simulink model "SimulationTest"  (R2025a)
settings: Solver=ode45  StartTime=0.0  StopTime=100  FixedStep=0.01  MaxStep=0.01  MinStep=0.001  RelTol=1e-3
model workspace (MAT data in the model file):
  L = 0.25
  R = 0.05
libraries: simulink x3, slpidlib x1
settings Model: PacingRate=1000  Creator=levirogalla  LastModifiedBy=levirogalla

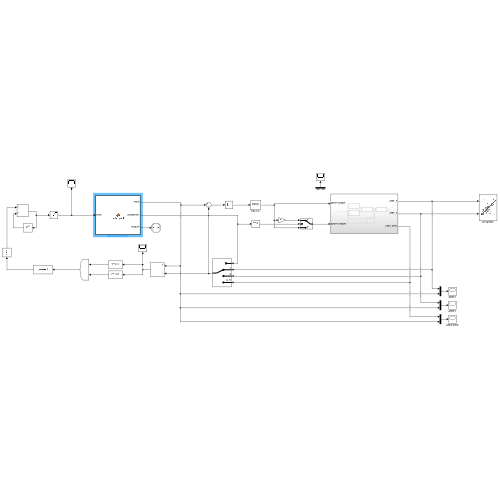
[thumbnail: Simulink's stored preview of the top-level diagram]
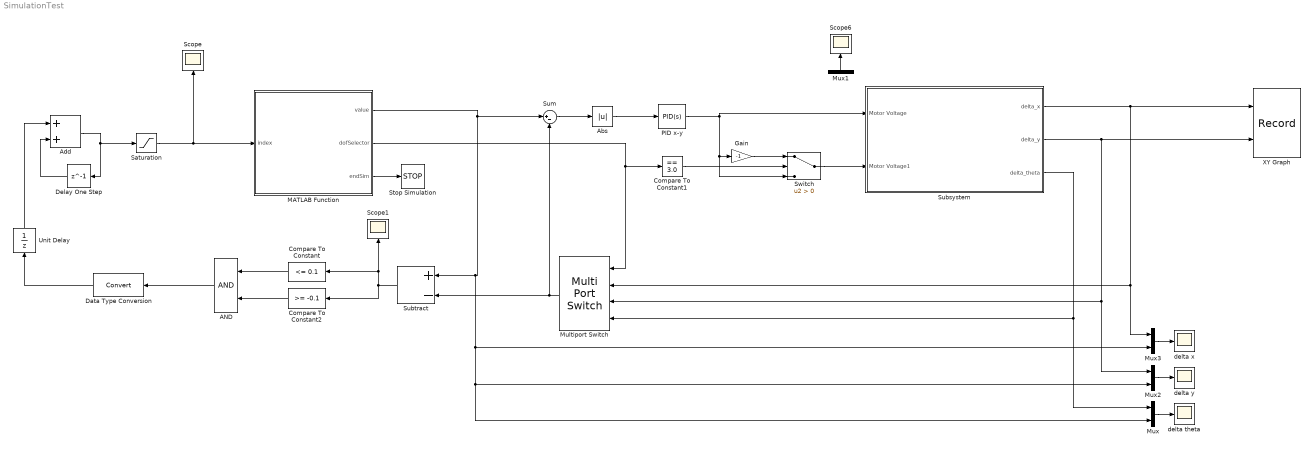
== system SimulationTest ==
  AND : Logic  IconShape=distinctive  AllPortsSameDT=off  OutDataTypeStr=boolean
  Abs : Abs  SaturateOnIntegerOverflow=off
  Add : Sum
  Compare To Constant : simulink/Logic and Bit Operations/Compare To Constant  relop=<=  const=0.1  OutDataTypeStr=boolean
  Compare To Constant1 : simulink/Logic and Bit Operations/Compare To Constant  relop===  const=3.0  OutDataTypeStr=boolean
  Compare To Constant2 : simulink/Logic and Bit Operations/Compare To Constant  relop=>=  const=-0.1  OutDataTypeStr=boolean
  Data Type Conversion : DataTypeConversion  SaturateOnIntegerOverflow=off  RndMeth=Floor
  Delay One Step : Delay  DelayLength=1
  Gain : Gain  Gain=-1
  MATLAB Function : MATLAB Function  TreatAsAtomicUnit=on
  Multiport Switch : MultiPortSwitch  SaturateOnIntegerOverflow=off  InputSameDT=off
  Mux{,1..3} (4 alike) : Mux  Inputs=2
  PID x-y : slpidlib/PID Controller  Controller=PID  Form=Parallel  TimeDomain=Continuous-time  UseExternalTs=off  SampleTime=-1  IntegratorMethod=Forward Euler  FilterMethod=Forward Euler  ControllerParametersSource=internal  P=0.25  I=0.001  UseKiTs=off  D=6.25  UseExternalDerivativeSource=off  N=100  UseFilter=on  TunerSelectOption=Transfer Function Based (PID Tuner App)  InitialConditionSource=internal  InitialConditionForIntegrator=0  InitialConditionForFilter=0  DifferentiatorICPrevScaledInput=0  ExternalReset=none  TrackingMode=off  Kt=1  LimitOutput=off  SatLimitsSource=internal  UpperSaturationLimit=50  LowerSaturationLimit=-inf  LinearizeAsGain=on  AntiWindupMode=none  Kb=1  LimitIntegrator=off  UpperIntegratorSaturationLimit=inf  LowerIntegratorSaturationLimit=-inf  POutMin=[]  POutMax=[]  IOutMin=[]  IOutMax=[]  DOutMin=[]  DOutMax=[]  NOutMin=[]  NOutMax=[]  SumOutMin=[]  SumOutMax=[]  SaturationOutMin=[]  SaturationOutMax=[]  PParamMin=[]  PParamMax=[]  IParamMin=[]  IParamMax=[]  DParamMin=[]  DParamMax=[]  NParamMin=[]  NParamMax=[]  KbParamMin=[]  KbParamMax=[]  KtParamMin=[]  KtParamMax=[]  KbOutMin=[]  KbOutMax=[]  KtOutMin=[]  KtOutMax=[]  IntegratorOutMin=[]  IntegratorOutMax=[]  FilterOutMin=[]  FilterOutMax=[]  SumI1OutMin=[]  SumI1OutMax=[]  SumI2OutMin=[]  SumI2OutMax=[]  SumI3OutMin=[]  SumI3OutMax=[]  SumI4OutMin=[]  SumI4OutMax=[]  SumDOutMin=[]  SumDOutMax=[]  DifferentiatorOutMin=[]  DifferentiatorOutMax=[]  FilterDiffOutCoefMin=[]  FilterDiffOutCoefMax=[]  ReciprocalOutMin=[]  ReciprocalOutMax=[]  SumDenOutMin=[]  SumDenOutMax=[]  SumNumOutMin=[]  SumNumOutMax=[]  DivideOutMin=[]  DivideOutMax=[]  UdiffTsProdOutMin=[]  UdiffTsProdOutMax=[]  NTsProdOutMin=[]  NTsProdOutMax=[]  UintegralTsProdOutMin=[]  UintegralTsProdOutMax=[]  UngainTsProdOutMin=[]  UngainTsProdOutMax=[]  ClampingZeroOutDataTypeStr=Inherit: Inherit via back propagation  ClampingZeroOutMin=[]  ClampingZeroOutMax=[]  FilterDenConstantOutDataTypeStr=Inherit: Inherit via back propagation  FilterDenConstantOutMin=[]  FilterDenConstantOutMax=[]  PCopyOutDataTypeStr=Inherit: Inherit via back propagation  PCopyOutMin=[]  PCopyOutMax=[]  NCopyOutDataTypeStr=Inherit: Inherit via back propagation  NCopyOutMin=[]  NCopyOutMax=[]  IntegratorContinuousStateAttributes=''  IntegratorStateMustResolveToSignalObject=off  IntegratorRTWStateStorageClass=Auto  FilterContinuousStateAttributes=''  FilterStateMustResolveToSignalObject=off  FilterRTWStateStorageClass=Auto  ParallelPVariant=InternalParameters  IdealPVariant=Disabled  IVariant=InternalParameters  DVariant=InternalParameters  IntegratorVariant=Continuous  SatVariant=Disabled  AWVariant=Passthrough  PCopyVariant=Disabled  TRVariant=Disabled  FdbkBlocksVariant=Forward  IdealPFdbkVariant=Disabled  SatFdbkVariant=Disabled  DerivativeFilterVariant=ContFilter  NVariant=InternalParameters  NCopyVariant=Disabled  FilterICVariant=InternalICsFilter  IntegratorICVariant=InternalICs  ExternalResetVariant=Disabled  TRSumVariant=Passthrough  SumFdbkVariant=Disabled  SumVariant=Sum_PID  TsampFilterVariant=InternalTs  TsampNgainVariant=Passthrough  TsampIntegralVariant=Disabled_SignalSpec  ExternalSaturationOutDataTypeStr=Inherit: Same as second input  DerivativeSourceVariant=ErrorSignal  PreIntVariant=InternalPreInt
  Saturation : Saturate  UpperLimit=5  LowerLimit=0  LinearizeAsGain=off
  Scope : Scope
      settings: ActiveDisplayYMinimum=-0.125  ActiveDisplayYMaximum=1.125
  Scope1 : Scope
      settings: ActiveDisplayYMinimum=-22.01338  ActiveDisplayYMaximum=19.1126  DataLoggingVariableName=ScopeData2
  Scope6 : Scope
      settings: ActiveDisplayYMinimum=-1208.50035  ActiveDisplayYMaximum=171.5621
  Stop Simulation : Stop
  Subsystem : Subsystem
  Subtract : Sum  Inputs=+-
  Sum : Sum  Inputs=|+-
  Switch : Switch  Criteria=u2 > Threshold  SaturateOnIntegerOverflow=off  InputSameDT=off
  Unit Delay : UnitDelay  SampleTime=-1  HasFrameUpgradeWarning=on
  XY Graph : Record  NumPorts=2.0  FileSettingsInternal="{\"entries\":[{\"content\":{\"excelSettings\":{\"content\":{},\"type\":\"Streamout.ExcelSettings\"},\"parquetSettings\":{\"content\":{},\"type\":\"Streamout.ParquetSettings\"}},\"type\":\"Streamout.FileSettingStorage\",\"uuid\":\"\"}],\"packageUris\":[\"http:\\/\\/schema.mathworks.com\\/mf0\\/streamout_blocks\\/R2020a\"],\"version\":\"1.0\"}"  FrameSettings=[0, 0]  Layout=[1 1]  SignalsInternal="{\"entries\":[{\"content\":{\"signals\":[{\"content\":{\"blockPath\":[],\"dimensions\":[1],\"domain\":\"\",\"lineColor\":\"#a2142f\",\"plots\":[ 1 ],\"port\":1,\"sid\":[\"\"],\"signalID\":1,\"signalName\":\"Subsystem:1\"},\"type\":\"RecordBlkView.Signal\",\"uuid\":\"\"},{\"content\":{\"blockPath\":[],\"dimensions\":[1],\"domain\":\"\",\"lineColor\":\"#139fff\",\"plots\":[ 1 ],\"port\":2,\"sid\":[\"\"],\"signalID\":2,\"signalName\":\"Subsystem:2\"},\"type\":\"RecordBlkView.Signal\",\"uuid\":\"\"}]},\"type\":\"RecordBlkView.InputSignals\",\"uuid\":\"\"}],\"packageUris\":[\"http:\\/\\/schema.mathworks.com\\/mf0\\/streamout_blocks\\/R2020a\"],\"version\":\"1.0\"}"  VisualizationBindings="{\"xyplotplugin\":{\"info\":[{\"series\":[{\"bindingParametersList\":[{\"parameter\":\"X-Axis\",\"signalID\":1,\"signalName\":\"Subsystem:1\"},{\"parameter\":\"Y-Axis\",\"signalID\":2,\"signalName\":\"Subsystem:2\"}],\"seriesID\":0}],\"subplotID\":1}]}}"  CompatibilityTag=XY
  delta theta : Scope
      settings: ActiveDisplayYMinimum=-12.11497  ActiveDisplayYMaximum=15.46071
  delta x : Scope
      settings: ActiveDisplayYMinimum=-13.25929  ActiveDisplayYMaximum=18.33365  DataLoggingVariableName=ScopeData2
  delta y : Scope
      settings: ActiveDisplayYMinimum=-13.32004  ActiveDisplayYMaximum=18.14667  DataLoggingVariableName=ScopeData3
  wires:
  Subsystem/2(delta_y) -> XY Graph/2, Mux2/1, Multiport Switch/3
  Subsystem/1(delta_x) -> XY Graph/1, Multiport Switch/2, Mux3/1
  Subsystem/3(delta_theta) -> Mux/1, Multiport Switch/4
  MATLAB Function/1(value) -> Sum/1, Mux/2, Mux2/2, Mux3/2, Subtract/1
  Multiport Switch/1 -> Subtract/2, Sum/2
  Add/1 -> Delay One Step/1, Saturation/1
  Delay One Step/1 -> Add/2
  MATLAB Function/2(dofSelector) -> Compare To Constant1/1, Multiport Switch/1
  Subtract/1 -> Compare To Constant2/1, Scope1/1, Compare To Constant/1
  Data Type Conversion/1 -> Unit Delay/1
  Saturation/1 -> MATLAB Function/1(index), Scope/1
  Unit Delay/1 -> Add/1
  Mux1/1 -> Scope6/1
  Compare To Constant2/1 -> AND/2
  Compare To Constant/1 -> AND/1
  AND/1 -> Data Type Conversion/1
  Compare To Constant1/1 -> Switch/2
  PID x-y/1 -> Subsystem/1(Motor Voltage), Switch/3, Gain/1
  Switch/1 -> Subsystem/2(Motor Voltage1)
  Gain/1 -> Switch/1
  Sum/1 -> Abs/1
  Abs/1 -> PID x-y/1
  Mux/1 -> delta theta/1
  Mux3/1 -> delta x/1
  Mux2/1 -> delta y/1
  MATLAB Function/3(endSim) -> Stop Simulation/1

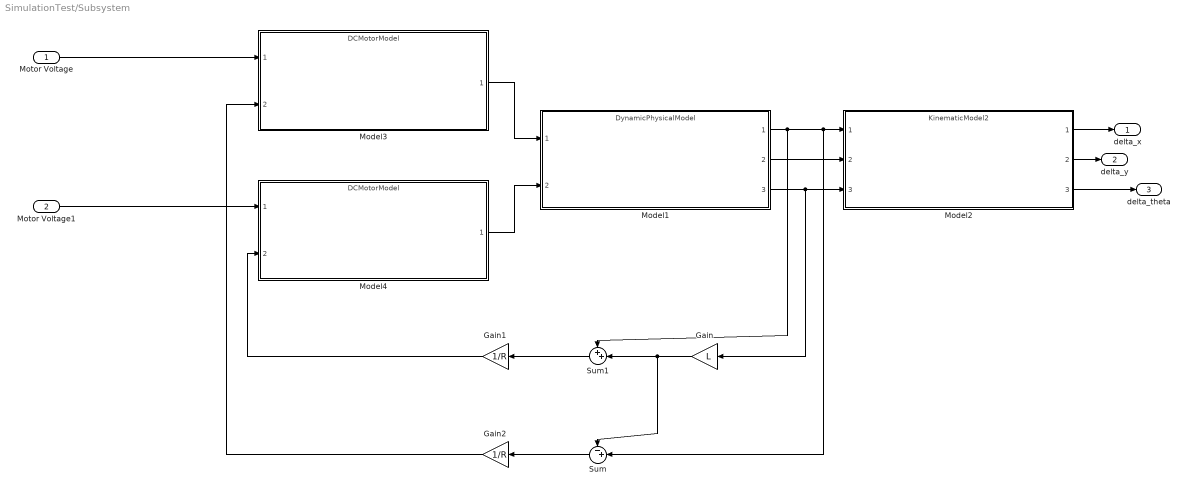
== system SimulationTest/Subsystem ==
  Motor Voltage : Inport
  Motor Voltage1 : Inport  Port=2
  Gain : Gain  Gain=L
  Gain1 : Gain  Gain=1/R
  Gain2 : Gain  Gain=1/R
  Model1 : ModelReference  ModelNameDialog=DynamicPhysicalModel.slx  SimulationMode=Normal  ModelReferenceVersion=3.1
  Model2 : ModelReference  ModelNameDialog=KinematicModel2.slx  SimulationMode=Normal  ModelReferenceVersion=3.1
  Model3 : ModelReference  ModelNameDialog=DCMotorModel.slx  SimulationMode=Normal  ModelReferenceVersion=3.1
  Model4 : ModelReference  ModelNameDialog=DCMotorModel.slx  SimulationMode=Normal  ModelReferenceVersion=3.1
  Sum : Sum  Inputs=-+|
  Sum1 : Sum  Inputs=++|
  delta_x : Outport
  delta_y : Outport  Port=2
  delta_theta : Outport  Port=3
  wires:
  Model1/1 -> Sum1/1, Sum/2, Model2/1
  Sum1/1 -> Gain1/1
  Gain/1 -> Sum/1, Sum1/2
  Model4/1 -> Model1/2
  Sum/1 -> Gain2/1
  Model1/2 -> Model2/2
  Model3/1 -> Model1/1
  Model1/3 -> Gain/1, Model2/3
  Gain2/1 -> Model3/2
  Gain1/1 -> Model4/2
  Motor Voltage1/1 -> Model4/1
  Model2/2 -> delta_y/1
  Model2/3 -> delta_theta/1
  Motor Voltage/1 -> Model3/1
  Model2/1 -> delta_x/1

== matlab function SimulationTest/MATLAB Function ==
  data: value output; dofSelector output; index input; endSim output
function [value, dofSelector, endSim] = pathSignal(index)
% Returns path values and a signal to stop simulation when out of bounds

% Define the path matrix
pathMatrix = [15, 1;
             -pi/2, 3;
             -10.1, 2;
             -pi, 3;
              6.9, 1
              -pi, 3];

% Get the size of the path
N = size(pathMatrix, 1);

% Initialize outputs
value = 0;
dofSelector = 1;
endSim = false;

% Check if index is within bounds
if index + 1 <= N
    value = pathMatrix(index + 1, 1);
    dofSelector = pathMatrix(index + 1, 2);
else
    endSim = true;  % signal to stop the simulation
end
